simulink model "multilevelinverter"  (Simulink 8.4)
settings: Solver=ode45  StartTime=0.0  StopTime=1  MaxStep=0.001  RelTol=1e-3
libraries: powerlib x19, simulink x10
settings Model: Creator=Muruganandham  LastModifiedBy=SELVA

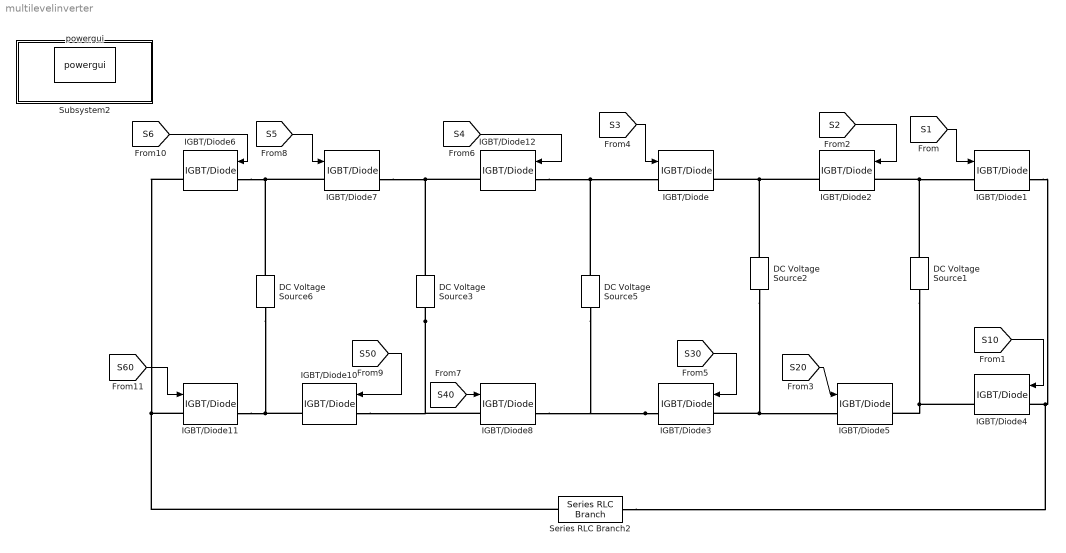
== system multilevelinverter ==
  DC Voltage Source{1..3,5..6} (5 alike) : powerlib/Electrical Sources/DC Voltage Source  Amplitude=66.5  Measurements=None
  IGBT/Diode{,1..8,10..12} (12 alike) : powerlib/Power Electronics/IGBT//Diode  Ron=1e-3  Rs=1e5  Cs=inf  Measurements=on
  Series RLC Branch2 : powerlib/Elements/Series RLC Branch  LConnTagsString=__new0  RConnTagsString=__new0  BranchType=R  Resistance=10  Inductance=1e-3  SetiL0=off  InitialCurrent=0  Capacitance=1e-6  Setx0=off  InitialVoltage=0  Measurements=None
  Subsystem2 : Subsystem  mask{fc=1000, m=1}
      mask prompts: fc "switching frequency"; m "modulation index"
  powergui : powerlib/powergui  Priority=1  SimulationMode=Discrete  SolverType=Tustin/Backward Euler (TBE)  SampleTime=50e-6  frequency=60  SPID=off  DisableSnubberDevices=off  DisableRonSwitches=off  DisableVfSwitches=off  SwTol=0  DisplayEquations=off  Interpol=off  methode=off  Ts=0  frequencyindice=0  Pbase=100e6  ErrMax=1e-4  Iterations=50  UnitsV=kV  UnitsW=MW  FunctionMessages=off  echomessages=off  HookPort=off  EnableUseOfTLC=off  x0status=blocks  RestoreLinks=warning  ResistiveCurrentMeasurement=off  Frange=[0:2:500]  Ylog=off  Xlog=on  ShowGrid=off  save=off  variable=ZData  structure=bh  ZoomFFT=off  StartTime=0.04  cycles=1  DisplayStyle=1  fundamental=50  FreqAxis=off  MaxFrequency=10000  frequencyindicesteady=1  RmsSteady=1  display=off
  wires:
  [S1] -> IGBT/Diode1/1
  [S10] -> IGBT/Diode4/1
  [S2] -> IGBT/Diode2/1
  [S20] -> IGBT/Diode5/1
  [S3] -> IGBT/Diode/1
  [S30] -> IGBT/Diode3/1
  [S40] -> IGBT/Diode8/1
  [S6] -> IGBT/Diode6/1
  [S4] -> IGBT/Diode12/1
  [S5] -> IGBT/Diode7/1
  [S50] -> IGBT/Diode10/1
  [S60] -> IGBT/Diode11/1
  connections:
  DC Voltage Source2/LConn1 -- IGBT/Diode2/RConn1 -- IGBT/Diode/RConn1
  DC Voltage Source1/RConn1 -- IGBT/Diode2/LConn1 -- IGBT/Diode1/LConn1
  DC Voltage Source2/RConn1 -- IGBT/Diode3/LConn1 -- IGBT/Diode5/LConn1
  DC Voltage Source1/LConn1 -- IGBT/Diode5/RConn1 -- IGBT/Diode4/RConn1
  IGBT/Diode1/RConn1 -- Series RLC Branch2/RConn1 -- IGBT/Diode4/LConn1
  DC Voltage Source6/RConn1 -- IGBT/Diode6/LConn1 -- IGBT/Diode7/LConn1
  DC Voltage Source3/LConn1 -- IGBT/Diode7/RConn1 -- IGBT/Diode12/RConn1
  DC Voltage Source6/LConn1 -- IGBT/Diode11/RConn1 -- IGBT/Diode10/RConn1
  DC Voltage Source3/RConn1 -- IGBT/Diode10/LConn1 -- IGBT/Diode8/LConn1
  IGBT/Diode12/LConn1 -- DC Voltage Source5/RConn1 -- IGBT/Diode/LConn1
  IGBT/Diode3/RConn1 -- IGBT/Diode8/RConn1 -- DC Voltage Source5/LConn1
  Series RLC Branch2/LConn1 -- IGBT/Diode11/LConn1 -- IGBT/Diode6/RConn1

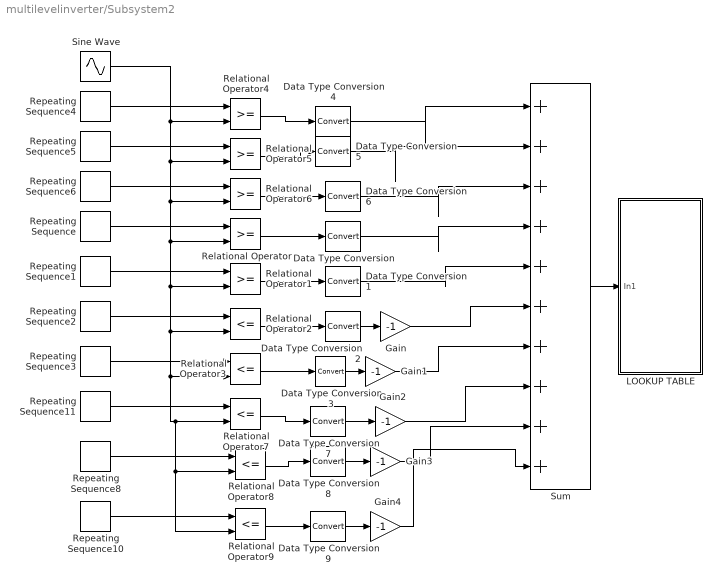
== system multilevelinverter/Subsystem2 ==
  Data Type Conversion{,1..9} (10 alike) : DataTypeConversion
  Gain{,1..4} (5 alike) : Gain  Gain=-1
  LOOKUP TABLE : Subsystem
  Relational Operator{,1,4..6} (5 alike) : RelationalOperator  OutDataTypeStr=boolean
  Relational Operator{2..3,7..9} (5 alike) : RelationalOperator  Operator=<=  OutDataTypeStr=boolean
  Repeating Sequence : simulink/Sources/Repeating Sequence  rep_seq_t="[0 (1/fc)/2  (1/fc)]"  rep_seq_y=[2 1 2]
  Repeating Sequence1 : simulink/Sources/Repeating Sequence  rep_seq_t="[0 (1/fc)/2  (1/fc)]"  rep_seq_y=[1 0 1]
  Repeating Sequence10 : simulink/Sources/Repeating Sequence  rep_seq_t="[0 (1/fc)/2  (1/fc)]"  rep_seq_y=[-5 -4 -5]
  Repeating Sequence11 : simulink/Sources/Repeating Sequence  rep_seq_t="[0 (1/fc)/2  (1/fc)]"  rep_seq_y=[-3 -2 -3]
  Repeating Sequence2 : simulink/Sources/Repeating Sequence  rep_seq_t="[0 (1/fc)/2  (1/fc)]"  rep_seq_y=[-1 0 -1]
  Repeating Sequence3 : simulink/Sources/Repeating Sequence  rep_seq_t="[0 (1/fc)/2  (1/fc)]"  rep_seq_y=[-2 -1 -2]
  Repeating Sequence4 : simulink/Sources/Repeating Sequence  rep_seq_t="[0 (1/fc)/2  (1/fc)]"  rep_seq_y=[4 5 4]
  Repeating Sequence5 : simulink/Sources/Repeating Sequence  rep_seq_t="[0 (1/fc)/2  (1/fc)]"  rep_seq_y=[4 3 4]
  Repeating Sequence6 : simulink/Sources/Repeating Sequence  rep_seq_t="[0 (1/fc)/2  (1/fc)]"  rep_seq_y=[3 2 3]
  Repeating Sequence8 : simulink/Sources/Repeating Sequence  rep_seq_t="[0 (1/fc)/2  (1/fc)]"  rep_seq_y=[-4 -3 -4]
  Sine Wave : Sin  Amplitude=5*m  Frequency=2*pi*50  SampleTime=0
  Sum : Sum  Inputs=|++++++++++
  wires:
  Data Type Conversion3/1 -> Gain1/1
  Data Type Conversion2/1 -> Gain/1
  Relational Operator3/1 -> Data Type Conversion3/1
  Relational Operator2/1 -> Data Type Conversion2/1
  Repeating Sequence3/1 -> Relational Operator3/1
  Repeating Sequence2/1 -> Relational Operator2/1
  Repeating Sequence1/1 -> Relational Operator1/1
  Repeating Sequence/1 -> Relational Operator/1
  Relational Operator1/1 -> Data Type Conversion1/1
  Relational Operator/1 -> Data Type Conversion/1
  Repeating Sequence6/1 -> Relational Operator6/1
  Repeating Sequence5/1 -> Relational Operator5/1
  Repeating Sequence4/1 -> Relational Operator4/1
  Relational Operator6/1 -> Data Type Conversion6/1
  Relational Operator5/1 -> Data Type Conversion5/1
  Relational Operator4/1 -> Data Type Conversion4/1
  Repeating Sequence8/1 -> Relational Operator8/1
  Repeating Sequence11/1 -> Relational Operator7/1
  Relational Operator9/1 -> Data Type Conversion9/1
  Relational Operator8/1 -> Data Type Conversion8/1
  Relational Operator7/1 -> Data Type Conversion7/1
  Data Type Conversion9/1 -> Gain4/1
  Data Type Conversion8/1 -> Gain3/1
  Data Type Conversion7/1 -> Gain2/1
  Repeating Sequence10/1 -> Relational Operator9/1
  Data Type Conversion4/1 -> Sum/1
  Data Type Conversion5/1 -> Sum/2
  Data Type Conversion6/1 -> Sum/3
  Data Type Conversion/1 -> Sum/4
  Data Type Conversion1/1 -> Sum/5
  Gain/1 -> Sum/6
  Gain1/1 -> Sum/7
  Gain2/1 -> Sum/8
  Gain3/1 -> Sum/9
  Gain4/1 -> Sum/10
  Sum/1 -> LOOKUP TABLE/1(In1)
  Sine Wave/1 -> Relational Operator5/2, Relational Operator6/2, Relational Operator/2, Relational Operator1/2, Relational Operator2/2, Relational Operator3/2, Relational Operator7/2, Relational Operator9/2, Relational Operator8/2, Relational Operator4/2

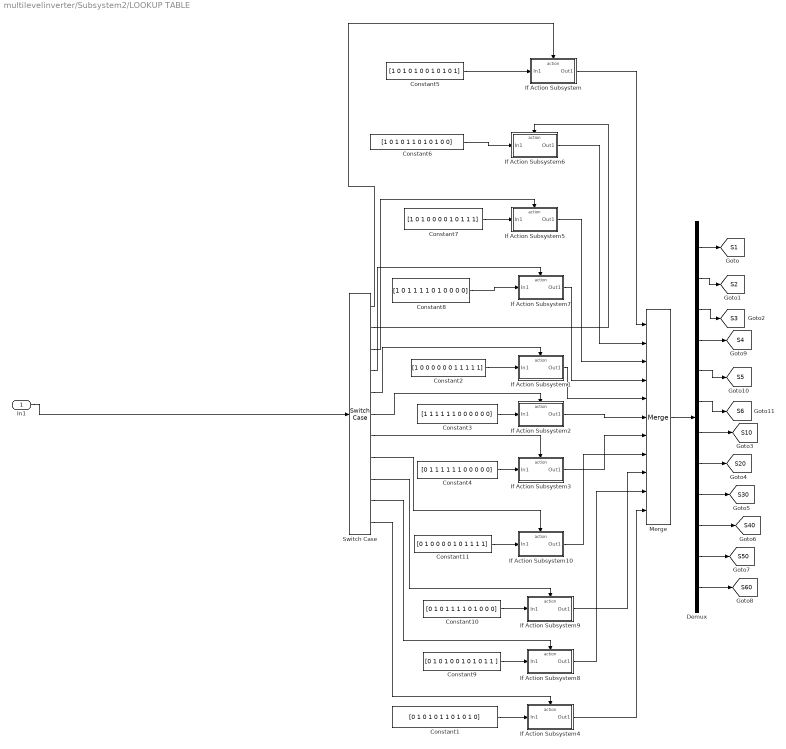
== system multilevelinverter/Subsystem2/LOOKUP TABLE ==
  In1 : Inport
  Constant1 : Constant  Value=[0 1 0 1 0 1 1 0 1 0 1 0]
  Constant10 : Constant  Value=[0 1 0 1 1 1 1 0 1 0 0 0]
  Constant11 : Constant  Value=[0 1 0 0 0 0 1 0 1 1 1 1]
  Constant2 : Constant  Value=[1 0 0 0 0 0 0 1 1 1 1 1]
  Constant3 : Constant  Value=[1 1 1 1 1 1 0 0 0 0 0 0]
  Constant4 : Constant  Value=[0 1 1 1 1 1 1 0 0 0 0 0]
  Constant5 : Constant  Value=[1 0 1 0 1 0 0 1 0 1 0 1]
  Constant6 : Constant  Value=[1 0 1 0 1 1 0 1 0 1 0 0]
  Constant7 : Constant  Value=[1 0 1 0 0 0 0 1 0 1 1 1]
  Constant8 : Constant  Value=[1 0 1 1 1 1 0 1 0 0 0 0]
  Constant9 : Constant  Value=[0 1 0 1 0 0 1 0 1 0 1 1 ]
  Demux : Demux  Outputs=12
  If Action Subsystem : Subsystem  TreatAsAtomicUnit=on
  If Action Subsystem1 : Subsystem  TreatAsAtomicUnit=on
  If Action Subsystem10 : Subsystem  TreatAsAtomicUnit=on
  If Action Subsystem2 : Subsystem  TreatAsAtomicUnit=on
  If Action Subsystem3 : Subsystem  TreatAsAtomicUnit=on
  If Action Subsystem4 : Subsystem  TreatAsAtomicUnit=on
  If Action Subsystem5 : Subsystem  TreatAsAtomicUnit=on
  If Action Subsystem6 : Subsystem  TreatAsAtomicUnit=on
  If Action Subsystem7 : Subsystem  TreatAsAtomicUnit=on
  If Action Subsystem8 : Subsystem  TreatAsAtomicUnit=on
  If Action Subsystem9 : Subsystem  TreatAsAtomicUnit=on
  Merge : Merge  Inputs=11
  Switch Case : SwitchCase  CaseConditions={-5 -4 -3 -2 -1 0 1 2 3 4 5}  ShowDefaultCase=off
  tag scope: S10=global, S1=global, S20=global, S2=global, S30=global, S3=global, S40=global, S4=global, S50=global, S5=global, S60=global, S6=global
  wires:
  Merge/1 -> Demux/1
  If Action Subsystem/1(Out1) -> Merge/1
  Constant4/1 -> If Action Subsystem3/1(In1)
  Constant3/1 -> If Action Subsystem2/1(In1)
  Constant2/1 -> If Action Subsystem1/1(In1)
  Switch Case/6 -> If Action Subsystem2/Action
  If Action Subsystem6/1(Out1) -> Merge/2
  If Action Subsystem5/1(Out1) -> Merge/3
  If Action Subsystem7/1(Out1) -> Merge/4
  If Action Subsystem1/1(Out1) -> Merge/5
  If Action Subsystem2/1(Out1) -> Merge/6
  If Action Subsystem3/1(Out1) -> Merge/7
  Constant9/1 -> If Action Subsystem8/1(In1)
  Constant10/1 -> If Action Subsystem9/1(In1)
  Constant11/1 -> If Action Subsystem10/1(In1)
  Switch Case/11 -> If Action Subsystem4/Action
  If Action Subsystem4/1(Out1) -> Merge/11
  Switch Case/10 -> If Action Subsystem8/Action
  Switch Case/9 -> If Action Subsystem9/Action
  Switch Case/8 -> If Action Subsystem10/Action
  Switch Case/7 -> If Action Subsystem3/Action
  Switch Case/5 -> If Action Subsystem1/Action
  Switch Case/4 -> If Action Subsystem7/Action
  Switch Case/3 -> If Action Subsystem5/Action
  Switch Case/2 -> If Action Subsystem6/Action
  Switch Case/1 -> If Action Subsystem/Action
  Constant6/1 -> If Action Subsystem6/1(In1)
  Constant7/1 -> If Action Subsystem5/1(In1)
  Constant8/1 -> If Action Subsystem7/1(In1)
  If Action Subsystem10/1(Out1) -> Merge/8
  If Action Subsystem9/1(Out1) -> Merge/9
  If Action Subsystem8/1(Out1) -> Merge/10
  Demux/3 -> [S3]
  Demux/2 -> [S2]
  Demux/1 -> [S1]
  Demux/7 -> [S10]
  Demux/8 -> [S20]
  Demux/9 -> [S30]
  Demux/10 -> [S40]
  Demux/11 -> [S50]
  Demux/12 -> [S60]
  Demux/6 -> [S6]
  Demux/5 -> [S5]
  Demux/4 -> [S4]
  Constant1/1 -> If Action Subsystem4/1(In1)
  Constant5/1 -> If Action Subsystem/1(In1)
  In1/1 -> Switch Case/1

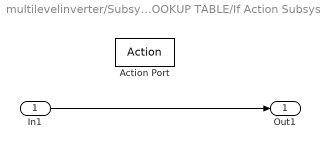
== system multilevelinverter/Subsystem2/LOOKUP TABLE/If Action Subsystem ==
  In1 : Inport
  Action Port : ActionPort  ActionType=case
  Out1 : Outport
  wires:
  In1/1 -> Out1/1

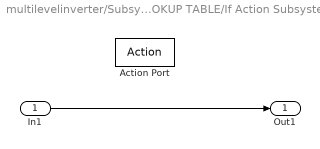
== system multilevelinverter/Subsystem2/LOOKUP TABLE/If Action Subsystem1 ==
  In1 : Inport
  Action Port : ActionPort  ActionType=case
  Out1 : Outport
  wires:
  In1/1 -> Out1/1

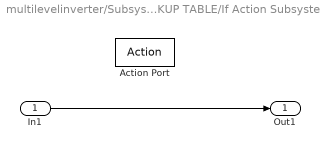
== system multilevelinverter/Subsystem2/LOOKUP TABLE/If Action Subsystem10 ==
  In1 : Inport
  Action Port : ActionPort  ActionType=case
  Out1 : Outport
  wires:
  In1/1 -> Out1/1

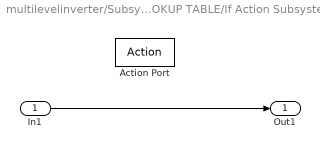
== system multilevelinverter/Subsystem2/LOOKUP TABLE/If Action Subsystem2 ==
  In1 : Inport
  Action Port : ActionPort  ActionType=case
  Out1 : Outport
  wires:
  In1/1 -> Out1/1

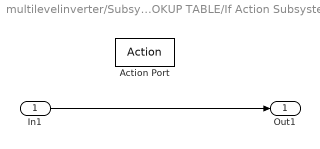
== system multilevelinverter/Subsystem2/LOOKUP TABLE/If Action Subsystem3 ==
  In1 : Inport
  Action Port : ActionPort  ActionType=case
  Out1 : Outport
  wires:
  In1/1 -> Out1/1

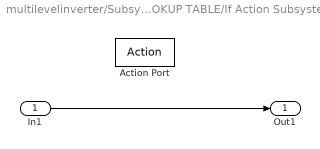
== system multilevelinverter/Subsystem2/LOOKUP TABLE/If Action Subsystem4 ==
  In1 : Inport
  Action Port : ActionPort  ActionType=case
  Out1 : Outport
  wires:
  In1/1 -> Out1/1

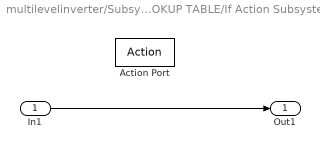
== system multilevelinverter/Subsystem2/LOOKUP TABLE/If Action Subsystem5 ==
  In1 : Inport
  Action Port : ActionPort  ActionType=case
  Out1 : Outport
  wires:
  In1/1 -> Out1/1

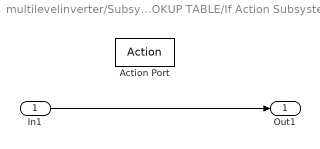
== system multilevelinverter/Subsystem2/LOOKUP TABLE/If Action Subsystem6 ==
  In1 : Inport
  Action Port : ActionPort  ActionType=case
  Out1 : Outport
  wires:
  In1/1 -> Out1/1

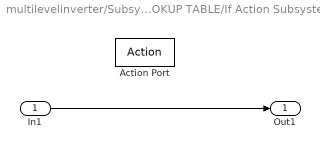
== system multilevelinverter/Subsystem2/LOOKUP TABLE/If Action Subsystem7 ==
  In1 : Inport
  Action Port : ActionPort  ActionType=case
  Out1 : Outport
  wires:
  In1/1 -> Out1/1

== system multilevelinverter/Subsystem2/LOOKUP TABLE/If Action Subsystem8 ==
  In1 : Inport
  Action Port : ActionPort  ActionType=case
  Out1 : Outport
  wires:
  In1/1 -> Out1/1

== system multilevelinverter/Subsystem2/LOOKUP TABLE/If Action Subsystem9 ==
  In1 : Inport
  Action Port : ActionPort  ActionType=case
  Out1 : Outport
  wires:
  In1/1 -> Out1/1
